simulink library "pwrsysVICtrl_202301"  (R2018a)
settings: Solver=VariableStepAuto  StartTime=0.0  StopTime=10.0  RelTol=1e-3
values from neighbouring files (symbols this model uses):
  Ts = 1e-6    (= 1e-06)    [SequenceSeparation_script.m]
undefined symbols (not defined in the file or in its folder): fn, Kp, Ti, Ts_control, Uabp, WT, X, zeta
libraries: pwrsysBasic x12, powerlib_meascontrol x8, pwrsysVICtrl x5, pwrsysTransf x1
settings Model: Creator=daniemot  LastModifiedBy=daniemot
settings OptimizationCC: LifeSpan=inf
settings DebuggingCC: SFExecutionAtInitializationDiag=none
settings CodeAppCC: StateflowObjectComments=on

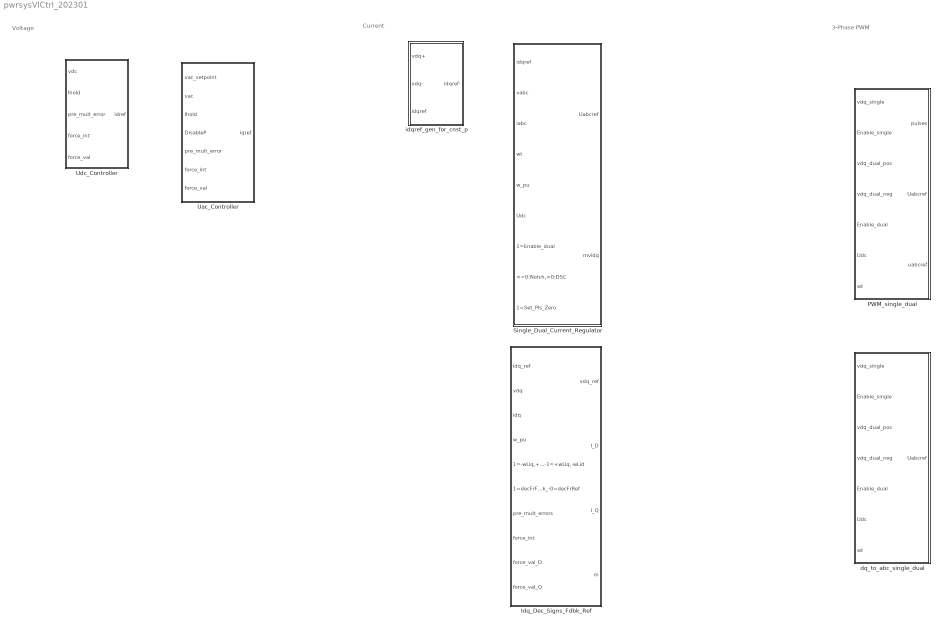
== system pwrsysVICtrl_202301 ==
  note: Voltage
  note: Current
  note: 3-Phase PWM
  Idq_Dec_Signs_Fdbk_Ref : Subsystem  mask(Idq Controller - PI regulator with anti-windup){Ts=Ts_control, fn=50, Kp=0.4, Ti=0.13, L=0.3, PI_max=1.5, PI_min=-1.5, TrafoPhaseComp=0}
      mask prompts: Ts "Sampling time [s]"; fn "Rated frequency: fn [Hz]"; Kp "Proportional gain: Kp [pu]"; Ti "Integral time: Ti [s]"; L "DQ decoupl. inductance: L [pu]"; PI_max "Maximum output [pu]"; PI_min "Minimum output [pu]"; TrafoPhaseComp "Transformer phase compensation [rad]"
      mask help:
      | Idq Controller
      | Discrete PI regulator with forward Euler approximation for the integrator.
      | Transfer function: 	Kp (1 + sTi) / (sTi)
      | The anti-windup freezes the integrator if the unlimited output of the PI goes beyond the limits.
      |
      | Phase compensation for transformer winding: PhaseTrafoComp
  PWM_single_dual : Subsystem  mask(Scaling of vdq ref and PWM gate generation){fsw=50, Ts=1/200000, Uabp=1000, PWM_Ini_Phase=90}
      mask prompts: fsw "Switching frequency [Hz]"; Ts "Sampling time [s]"; Uabp "Rated peak line voltage [V]"; PWM_Ini_Phase "PWM carrier initial phase [degrees]"
      mask help:
      | Scales vdq_ref by: U_line_peak / Udc
      |
      | Add third harmonic to uabc_ref for overmodulation
  Single_Dual_Current_Regulator : Subsystem  mask(Notch based dual dq current regulator){Ts=Ts_control, fgrid=fn, PI_X=X, PI_max=1.5, PI_min=-1.5, PWM_Uabp=Uabp, zetanotch=zeta, flpf=zeta, PI_Kp_single=Kp, PI_Ti_single=Ti, PI_Kp_dual=Kp, PI_Ti_dual=Ti}
      mask prompts: Ts "Sampling time controller [s]"; fgrid "Grid frequency [Hz]"; PI_X "Decoupling reactance X [pu]"; PI_max "PI max [pu]"; PI_min "PI min [pu]"; PWM_Uabp "Rated peak line voltage [V]"; zetanotch "Damping notch filters"; flpf "Cut-out frequelcy LPF noise [Hz]"; PI_Kp_single "Proportional gain Kp [pu/pu]"; PI_Ti_single "Integrator time Ti [s]"; PI_Kp_dual "Proportional gain Kp [pu/pu]"; PI_Ti_dual "Integrator time Ti [s]"
      mask help: To be used with "abc -> dq" and "acb -> dq" transformations. When va = V sin (wt), vb = V sin (wt-120), vc = V sin (wt+120), -> vd = V vq=0.
      mask DialogControl Container2 Prompt: Transducers
      mask DialogControl Container7 Prompt: PI regulator - Single
      mask DialogControl Container7_copy Prompt: PI regulator - Dual
  Uac_Controller : Subsystem  mask(Udc Controller - PI regulator with anti-windup){Ts=Ts_control, Kg=1, Kp=WT.LSC.Kp, Ti=WT.LSC.Ti, PI_max=1.5, PI_min=-1.5}
      mask prompts: Ts "Sampling time [s]"; Kg "Loop gain: Kg [pu]"; Kp "Proportional gain: Kp [pu]"; Ti "Integral time: Ti [s]"; PI_max "Maximum output [pu]"; PI_min "Minimum output [pu]"
      mask help:
      | Udc Controller
      | Discrete PI regulator with forward Euler approximation for the integrator.
      | Transfer function: 	Kp (1 + sTi) / (sTi)
      | The anti-windup freezes the integrator if the unlimited output of the PI goes beyond the limits.
  Udc_Controller : Subsystem  mask(Udc Controller - PI regulator with anti-windup){Ts=Ts_control, Kp=WT.LSC.Kp, Ti=WT.LSC.Ti, PI_max=1.5, PI_min=-1.5}
      mask prompts: Ts "Sampling time [s]"; Kp "Proportional gain: Kp [pu]"; Ti "Integral time: Ti [s]"; PI_max "Maximum output [pu]"; PI_min "Minimum output [pu]"
      mask help:
      | Udc Controller
      | Discrete PI regulator with forward Euler approximation for the integrator.
      | Transfer function: 	Kp (1 + sTi) / (sTi)
      | The anti-windup freezes the integrator if the unlimited output of the PI goes beyond the limits.
  dq_to_abc_single_dual : Subsystem  mask(Scaling of vdq ref and PWM gate generation){Ts=1/200000, Uabp=1000}
      mask prompts: Ts "Sampling time [s]"; Uabp "Rated peak line voltage [V]"
      mask help:
      | Scales vdq_ref by: U_line_peak / Udc
      |
      | Add third harmonic to uabc_ref for overmodulation
  idqref_gen_for_cnst_p : Subsystem  mask(Negative sequence current reference calculation){Ts_control=Ts_control}
      mask prompts: Ts_control "Sampling time [s]"
      mask help: Calculation of the negative sequence current references for removing active power second harmonic oscillations when in the presence of unbalanced voltages.
      mask Help:
      | Calculation of the negative sequence current references for removing active power second harmonic oscillations when in the presence of unbalanced voltages.
      | 
      | Second harmonic in instataneous reactive power will be increased as a result of the removal of the second harmonic in the active power.
      | 
      | To be used with "abc -> dq" and "acb -> dq" transformations. When va = V sin (wt), vb = V sin (wt-120), vc = V sin (wt+120), -> vd = V vq=0.
      | 
      | In "expanded" matrix form:
      | 	| idn | = - | -vdp  +vqp |^{-1} * | -vdn  +vqn | * | idp |
      | 	| iqn | =   | +vqp  +vdp |        | +vqn  +vdn |   | idq |
      | 
      | In matrix form
      | 	idqn  = - vdqp^{-1} * vdqn * idqp
      | 
      | Derived independently from, but later noticed that it was proposed by Chaudhary in 2012 at "Negative Sequence Current Control in Wind Power Plants With VSC-HVDC Connection", see eq. (11).
      | 
      | This block does not work for "abc (-omega) -> dq" (the formulation of Chaudhary 2012).

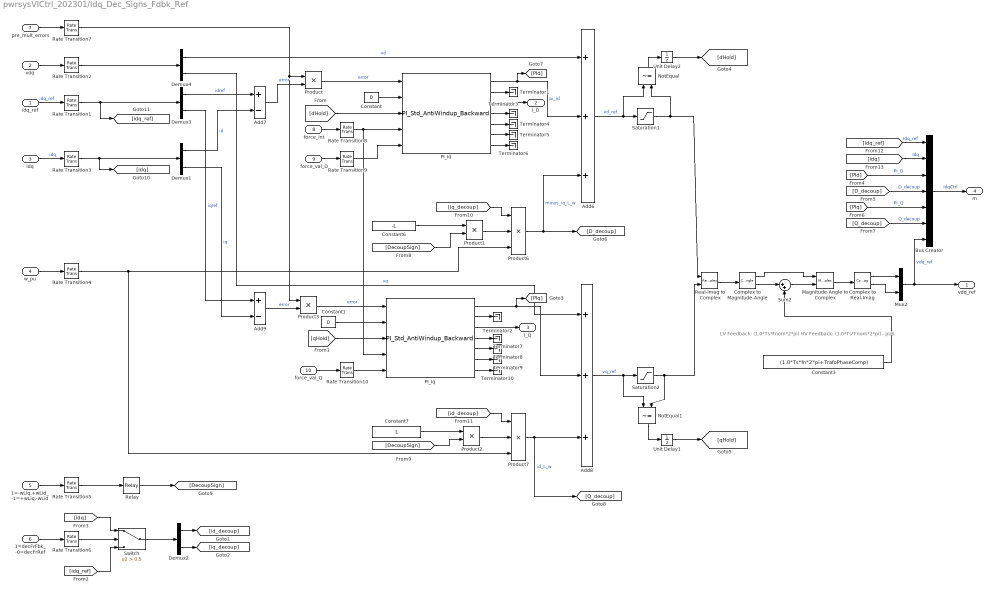
== system pwrsysVICtrl_202301/Idq_Dec_Signs_Fdbk_Ref ==
  note: LV Feedback: (1.0*Ts*Fnom*2*pi)
      | HV Feedback: (1.0*Ts*Fnom*2*pi) - pi/6
  idq_ref : Inport
  vdq : Inport  Port=2
  idq : Inport  Port=3
  w_pu : Inport  Port=4
  1=-wLiq,+wLid_-1=+wLiq,-wLid : Inport  Port=5
  1=decFrFbk_-0=decFrRef : Inport  Port=6
  pre_mult_errors : Inport  Port=7
  force_int : Inport  Port=8
  force_val_D : Inport  Port=9
  force_val_Q : Inport  Port=10
  Add6 : Sum  Inputs=+++
  Add7 : Sum  Inputs=+-
  Add8 : Sum  Inputs=+++
  Add9 : Sum  Inputs=+-
  Bus Creator : BusCreator  Inputs=7
  Complex to Magnitude-Angle : ComplexToMagnitudeAngle
  Complex to Real-Imag : ComplexToRealImag
  Constant : Constant  Value=0  SampleTime=Ts
  Constant1 : Constant  Value=0  SampleTime=Ts
  Constant3 : Constant  Value=(1.0*Ts*fn*2*pi+TrafoPhaseComp)  SampleTime=Ts
  Constant6 : Constant  Value=-L  SampleTime=Ts
  Constant7 : Constant  Value=L  SampleTime=Ts
  Demux{1..4} (4 alike) : Demux  Outputs=2
  Magnitude-Angle to Complex : MagnitudeAngleToComplex
  Mux2 : Mux  Inputs=2
  NotEqual : RelationalOperator  Operator=~=  OutDataTypeStr=boolean  RndMeth=Nearest
  NotEqual1 : RelationalOperator  Operator=~=  OutDataTypeStr=boolean  RndMeth=Nearest
  PI_Id : pwrsysBasic/PI_Std_AntiWindup_Backward  Ts=Ts  Kg=Kp  Kp=1  Ti=Ti  outMax=PI_max  outMin=PI_min
      settings: SourceProductName=NTNU Power Systems
  PI_Iq : pwrsysBasic/PI_Std_AntiWindup_Backward  Ts=Ts  Kg=Kp  Kp=1  Ti=Ti  outMax=PI_max  outMin=PI_min
      settings: SourceProductName=NTNU Power Systems
  Product : Product
  Product1 : Product  RndMeth=Zero
  Product2 : Product  RndMeth=Zero
  Product3 : Product
  Product6 : Product  Inputs=3  RndMeth=Zero
  Product7 : Product  Inputs=3  RndMeth=Zero
  Rate Transition1 : RateTransition  InitialCondition=[0 0]  OutPortSampleTime=Ts
  Rate Transition{6..10} (5 alike) : RateTransition  OutPortSampleTime=Ts
  Rate Transition2 : RateTransition  InitialCondition=[0 0]  OutPortSampleTime=Ts
  Rate Transition3 : RateTransition  InitialCondition=[0 0]  OutPortSampleTime=Ts
  Rate Transition4 : RateTransition  InitialCondition=1  OutPortSampleTime=Ts
  Rate Transition5 : RateTransition  InitialCondition=1  OutPortSampleTime=Ts
  Real-Imag to Complex : RealImagToComplex
  Relay : Relay  OnSwitchValue=0  OffSwitchValue=-0.1  OffOutputValue=-1
  Saturation1 : Saturate  UpperLimit=PI_max  LowerLimit=PI_min
  Saturation2 : Saturate  UpperLimit=PI_max  LowerLimit=PI_min
  Sum2 : Sum  Inputs=|++
  Switch : Switch  Criteria=u2 > Threshold  Threshold=0.5
  Terminator{1..10} (10 alike) : Terminator
  Unit Delay1 : UnitDelay  SampleTime=Ts
  Unit Delay2 : UnitDelay  SampleTime=Ts
  vdq_ref : Outport
  I_D : Outport  Port=2
  I_Q : Outport  Port=3
  m : Outport  Port=4
  wires:
  w_pu/1 -> Rate Transition4/1
  Product3/1 -> PI_Iq/1  "error"
  PI_Id/1 -> Add6/2, [PId]  "pi_id"
  Constant6/1 -> Product1/1
  Constant7/1 -> Product2/1
  Demux1/1 -> Add7/2  "id"
  Product7/1 -> [Q_decoup], Add8/3  "id_L_w"
  Demux4/1 -> Add6/1  "vd"
  Product/1 -> PI_Id/1  "error"
  Demux1/2 -> Add9/2  "iq"
  Product6/1 -> Add6/3, [D_decoup]  "minus_iq_L_w"
  Demux4/2 -> Add8/1  "vq"
  Mux2/1 -> Bus Creator/7, vdq_ref/1  "vdq_ref"
  idq/1 -> Rate Transition3/1  "idq"
  vdq/1 -> Rate Transition2/1
  Add8/1 -> NotEqual1/1, Saturation2/1  "vq_ref"
  Add6/1 -> NotEqual/1, Saturation1/1  "vd_ref"
  idq_ref/1 -> Rate Transition1/1  "idq_ref"
  Demux3/1 -> Add7/1  "idref"
  Demux3/2 -> Add9/1  "iqref"
  Magnitude-Angle to Complex/1 -> Complex to Real-Imag/1
  Real-Imag to Complex/1 -> Complex to Magnitude-Angle/1
  Complex to Magnitude-Angle/1 -> Magnitude-Angle to Complex/1
  Complex to Magnitude-Angle/2 -> Sum2/1
  Sum2/1 -> Magnitude-Angle to Complex/2
  Constant3/1 -> Sum2/2
  Complex to Real-Imag/1 -> Mux2/1
  Complex to Real-Imag/2 -> Mux2/2
  [PId] -> Bus Creator/3  "PI_D"
  [D_decoup] -> Bus Creator/4  "D_decoup"
  [PIq] -> Bus Creator/5  "PI_Q"
  Bus Creator/1 -> m/1  "IdqCtrl"
  [Q_decoup] -> Bus Creator/6  "Q_decoup"
  Saturation1/1 -> NotEqual/2, Real-Imag to Complex/1
  NotEqual/1 -> Unit Delay2/1
  Saturation2/1 -> NotEqual1/2, Real-Imag to Complex/2
  NotEqual1/1 -> Unit Delay1/1
  Unit Delay2/1 -> [dHold]
  Unit Delay1/1 -> [qHold]
  [dHold] -> PI_Id/3
  [qHold] -> PI_Iq/3
  Relay/1 -> [DecoupSign]
  1=-wLiq,+wLid_-1=+wLiq,-wLid/1 -> Rate Transition5/1
  [DecoupSign] -> Product1/2
  Product1/1 -> Product6/2
  Product2/1 -> Product7/2
  [DecoupSign] -> Product2/2
  [idq_ref] -> Switch/3
  Demux2/2 -> [iq_decoup]
  1=decFrFbk_-0=decFrRef/1 -> Rate Transition6/1
  Demux2/1 -> [id_decoup]
  Switch/1 -> Demux2/1
  [idq] -> Switch/1
  [iq_decoup] -> Product6/1
  [id_decoup] -> Product7/1
  [idq_ref] -> Bus Creator/1  "Idq_ref"
  [idq] -> Bus Creator/2  "Idq"
  force_int/1 -> Rate Transition8/1
  force_val_D/1 -> Rate Transition9/1
  force_val_Q/1 -> Rate Transition10/1
  Add9/1 -> Product3/2  "error"
  Add7/1 -> Product/2  "error"
  pre_mult_errors/1 -> Rate Transition7/1
  PI_Id/3 -> I_D/1
  Constant/1 -> PI_Id/2
  PI_Id/2 -> Terminator1/1
  PI_Id/4 -> Terminator3/1
  PI_Id/5 -> Terminator4/1
  PI_Id/6 -> Terminator5/1
  PI_Id/7 -> Terminator6/1
  PI_Iq/2 -> Terminator2/1
  PI_Iq/4 -> Terminator7/1
  PI_Iq/5 -> Terminator8/1
  PI_Iq/6 -> Terminator9/1
  PI_Iq/7 -> Terminator10/1
  PI_Iq/3 -> I_Q/1
  PI_Iq/1 -> Add8/2, [PIq]
  Constant1/1 -> PI_Iq/2
  Rate Transition2/1 -> Demux4/1
  Rate Transition1/1 -> [idq_ref], Demux3/1
  Rate Transition3/1 -> Demux1/1, [idq]
  Rate Transition4/1 -> Product7/3, Product6/3
  Rate Transition5/1 -> Relay/1
  Rate Transition6/1 -> Switch/2
  Rate Transition7/1 -> Product3/1, Product/1
  Rate Transition8/1 -> PI_Iq/4, PI_Id/4
  Rate Transition9/1 -> PI_Id/5
  Rate Transition10/1 -> PI_Iq/5

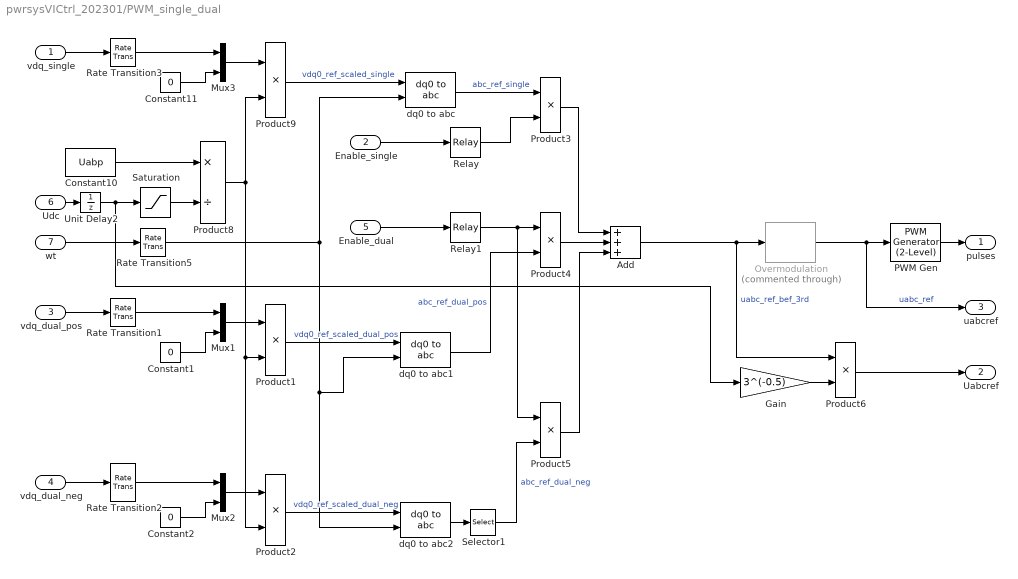
== system pwrsysVICtrl_202301/PWM_single_dual ==
  vdq_single : Inport
  Enable_single : Inport  Port=2
  vdq_dual_pos : Inport  Port=3
  vdq_dual_neg : Inport  Port=4
  Enable_dual : Inport  Port=5
  Udc : Inport  Port=6
  wt : Inport  Port=7
  Add : Sum  Inputs=+++
  Constant1 : Constant  Value=0
  Constant10 : Constant  Value=Uabp
  Constant11 : Constant  Value=0
  Constant2 : Constant  Value=0
  Gain : Gain  Gain=3^(-0.5)
  Mux1 : Mux  Inputs=[2 1]
  Mux2 : Mux  Inputs=[2 1]
  Mux3 : Mux  Inputs=[2 1]
  Overmodulation : powerlib_meascontrol/Pulse & Signal Generators/Overmodulation  Commented=through  OverModType=Third harmonic
      settings: SourceProductName=Simscape Power Systems  SourceProductBaseCode=PS
  PWM Gen : powerlib_meascontrol/Pulse & Signal Generators/PWM Generator (2-Level)  ModulatorType=Three-phase bridge (6 pulses)  ModulatorMode=Unsynchronized  Fc=fsw  Pc=PWM_Ini_Phase  nF=27  MinMax="[ -1  1 ]"  SamplingTechnique=Asymmetrical regular (double edge)  ModulatingSignals=off  m=0.8  Freq=60  Phase=0  Ts=Ts  ShowCarrierOutport=off
      settings: SourceProductName=Simscape Power Systems
  Product{1..6,9} (7 alike) : Product  Inputs=**
  Product8 : Product  Inputs=*/
  Rate Transition{1..3,5} (4 alike) : RateTransition  OutPortSampleTime=Ts
  Relay : Relay  OnSwitchValue=0.6  OffSwitchValue=0.4
  Relay1 : Relay  OnSwitchValue=0.6  OffSwitchValue=0.4
  Saturation : Saturate  UpperLimit=10*Uabp  LowerLimit=0.001*Uabp
  Selector1 : Selector  InputPortWidth=3  IndexOptions=Index vector (dialog)  Indices=[1 3 2]  OutputSizes=1
  Unit Delay2 : UnitDelay  InitialCondition=Uabp  SampleTime=Ts
  dq0 to abc : powerlib_meascontrol/Transformations/dq0 to abc  Alignment=90 degrees behind phase A axis
  dq0 to abc1 : powerlib_meascontrol/Transformations/dq0 to abc  Alignment=90 degrees behind phase A axis
  dq0 to abc2 : powerlib_meascontrol/Transformations/dq0 to abc  Alignment=90 degrees behind phase A axis
  pulses : Outport
  Uabcref : Outport  Port=2
  uabcref : Outport  Port=3
  wires:
  dq0 to abc1/1 -> Product4/2  "abc_ref_dual_pos"
  Rate Transition5/1 -> dq0 to abc/2, dq0 to abc1/2, dq0 to abc2/2
  Product1/1 -> dq0 to abc1/1  "vdq0_ref_scaled_dual_pos"
  vdq_dual_pos/1 -> Rate Transition1/1
  Constant1/1 -> Mux1/2
  Mux1/1 -> Product1/1
  Rate Transition1/1 -> Mux1/1
  Product6/1 -> Uabcref/1
  vdq_single/1 -> Rate Transition3/1
  PWM Gen/1 -> pulses/1
  Udc/1 -> Unit Delay2/1
  Overmodulation/1 -> uabcref/1, PWM Gen/1  "uabc_ref"
  Constant10/1 -> Product8/1
  wt/1 -> Rate Transition5/1
  Rate Transition3/1 -> Mux3/1
  Mux3/1 -> Product9/1
  Unit Delay2/1 -> Gain/1, Saturation/1
  Product9/1 -> dq0 to abc/1  "vdq0_ref_scaled_single"
  Constant11/1 -> Mux3/2
  dq0 to abc/1 -> Product3/1  "abc_ref_single"
  Enable_single/1 -> Relay/1
  Enable_dual/1 -> Relay1/1
  Add/1 -> Product6/1, Overmodulation/1  "uabc_ref_bef_3rd"
  Saturation/1 -> Product8/2
  Product8/1 -> Product2/2, Product1/2, Product9/2
  Rate Transition2/1 -> Mux2/1
  vdq_dual_neg/1 -> Rate Transition2/1
  Mux2/1 -> Product2/1
  Constant2/1 -> Mux2/2
  Product2/1 -> dq0 to abc2/1  "vdq0_ref_scaled_dual_neg"
  dq0 to abc2/1 -> Selector1/1
  Selector1/1 -> Product5/2  "abc_ref_dual_neg"
  Relay/1 -> Product3/2
  Product3/1 -> Add/1
  Product4/1 -> Add/2
  Relay1/1 -> Product5/1, Product4/1
  Product5/1 -> Add/3
  Gain/1 -> Product6/2

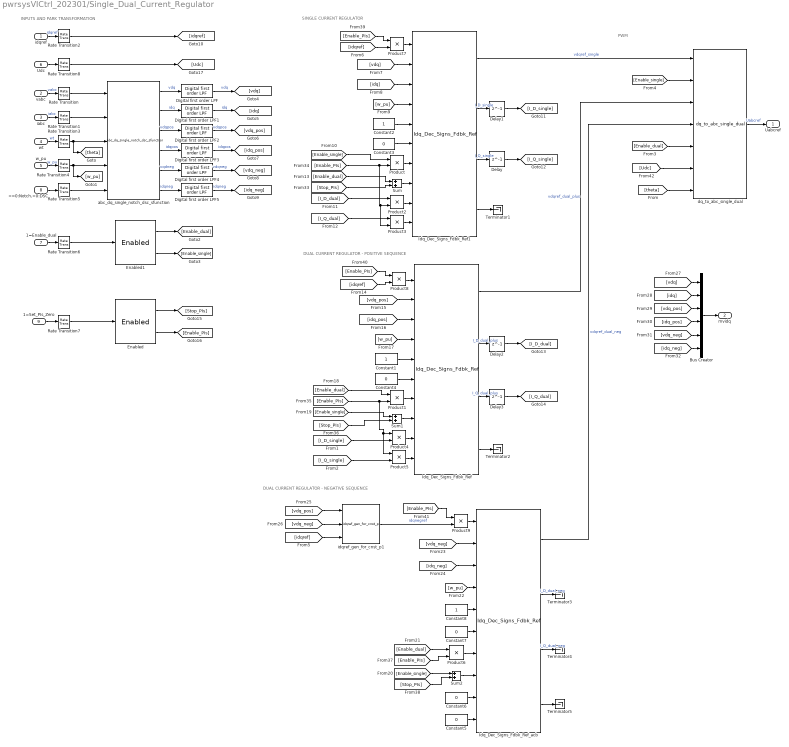
== system pwrsysVICtrl_202301/Single_Dual_Current_Regulator ==
  note: INPUTS AND PARK TRANSFORMATION
  note: SINGLE CURRENT REGULATOR
  note: DUAL CURRENT REGULATOR - POSITIVE SEQUENCE
  note: DUAL CURRENT REGULATOR - NEGATIVE SEQUENCE
  note: PWM
  idqref : Inport
  vabc : Inport  Port=2
  iabc : Inport  Port=3
  wt : Inport  Port=4
  w_pu : Inport  Port=5
  Udc : Inport  Port=6
  1=Enable_dual : Inport  Port=7
  <=0:Notch,>0:DSC : Inport  Port=8
  1=Set_PIs_Zero : Inport  Port=9
  Bus Creator : BusCreator  Inputs=6
  Constant1 : Constant  SampleTime=Ts
  Constant2 : Constant  SampleTime=Ts
  Constant{3..7} (5 alike) : Constant  Value=0  SampleTime=Ts
  Constant8 : Constant  SampleTime=Ts
  Delay{,1..3} (4 alike) : Delay  DelayLength=1  InitialCondition=0  SampleTime=Ts
  Digital first order LPF{,1..5} (6 alike) : pwrsysBasic/Digital first order LPF  Ts=Ts  fcutout=flpf
      settings: SourceProductName=NTNU Power Systems
  Enabled : pwrsysBasic/Enabled
      settings: SourceProductName=NTNU Power Systems
  Enabled1 : pwrsysBasic/Enabled
      settings: SourceProductName=NTNU Power Systems
  Idq_Dec_Signs_Fdbk_Ref : pwrsysVICtrl/Idq_Dec_Signs_Fdbk_Ref  Ts=Ts  fn=fgrid  Kp=PI_Kp_dual  Ti=PI_Ti_dual  L=PI_X  PI_max=PI_max  PI_min=PI_min  TrafoPhaseComp=0
      settings: SourceProductName=NTNU Power Systems
  Idq_Dec_Signs_Fdbk_Ref1 : pwrsysVICtrl/Idq_Dec_Signs_Fdbk_Ref  Ts=Ts  fn=fgrid  Kp=PI_Kp_single  Ti=PI_Ti_single  L=PI_X  PI_max=PI_max  PI_min=PI_min  TrafoPhaseComp=0
      settings: SourceProductName=NTNU Power Systems
  Idq_Dec_Signs_Fdbk_Ref_acb : pwrsysVICtrl/Idq_Dec_Signs_Fdbk_Ref  Ts=Ts  fn=fgrid  Kp=PI_Kp_dual  Ti=PI_Ti_dual  L=PI_X  PI_max=PI_max  PI_min=PI_min  TrafoPhaseComp=0
      settings: SourceProductName=NTNU Power Systems
  Product{,1..9} (10 alike) : Product
  Rate Transition : RateTransition  InitialCondition=[0 0 0]  OutPortSampleTime=Ts
  Rate Transition1 : RateTransition  InitialCondition=[0 0 0]  OutPortSampleTime=Ts
  Rate Transition2 : RateTransition  InitialCondition=[0 0]  OutPortSampleTime=Ts
  Rate Transition{3,5..7} (4 alike) : RateTransition  OutPortSampleTime=Ts
  Rate Transition4 : RateTransition  InitialCondition=1  OutPortSampleTime=Ts
  Rate Transition8 : RateTransition  InitialCondition=1  OutPortSampleTime=Ts
  Sum : Sum
  Sum1 : Sum
  Sum2 : Sum
  Terminator{1..5} (5 alike) : Terminator
  abc_dq_single_notch_dsc_sfunction : pwrsysTransf/abc_dq_single_notch_dsc_sfunction  Ts=Ts  fn=2*fgrid  zeta=zetanotch
      settings: SourceProductName=NTNU Power Systems
  dq_to_abc_single_dual : pwrsysVICtrl/dq_to_abc_single_dual  Ts=Ts  Uabp=PWM_Uabp
      settings: SourceProductName=NTNU Power Systems
  idqref_gen_for_cnst_p1 : pwrsysVICtrl/idqref_gen_for_cnst_p  Ts_control=Ts
      settings: SourceProductName=NTNU Power Systems
  Uabcref : Outport
  mvidq : Outport  Port=2
  wires:
  1=Enable_dual/1 -> Rate Transition6/1
  Enabled1/2 -> [Enable_single]
  Enabled1/1 -> [Enable_dual]
  1=Set_PIs_Zero/1 -> Rate Transition7/1
  Product9/1 -> Idq_Dec_Signs_Fdbk_Ref_acb/1
  [Enable_PIs] -> Product9/1
  Product8/1 -> Idq_Dec_Signs_Fdbk_Ref/1
  [Enable_PIs] -> Product8/1
  Product7/1 -> Idq_Dec_Signs_Fdbk_Ref1/1
  [Enable_PIs] -> Product7/1
  Sum2/1 -> Idq_Dec_Signs_Fdbk_Ref_acb/8
  [Stop_PIs] -> Sum2/2
  Product6/1 -> Idq_Dec_Signs_Fdbk_Ref_acb/7
  [Enable_PIs] -> Product6/2
  Product4/1 -> Idq_Dec_Signs_Fdbk_Ref/9
  Product5/1 -> Idq_Dec_Signs_Fdbk_Ref/10
  [Stop_PIs] -> Sum1/2
  Sum1/1 -> Idq_Dec_Signs_Fdbk_Ref/8
  [Enable_PIs] -> Product1/2, Product4/1, Product5/1
  Product1/1 -> Idq_Dec_Signs_Fdbk_Ref/7
  Product2/1 -> Idq_Dec_Signs_Fdbk_Ref1/9
  [Stop_PIs] -> Sum/2
  Product3/1 -> Idq_Dec_Signs_Fdbk_Ref1/10
  Sum/1 -> Idq_Dec_Signs_Fdbk_Ref1/8
  Product/1 -> Idq_Dec_Signs_Fdbk_Ref1/7
  [Enable_PIs] -> Product/2, Product2/2, Product3/2
  Enabled/2 -> [Enable_PIs]
  Enabled/1 -> [Stop_PIs]
  [idq_neg] -> Bus Creator/6
  [vdq_neg] -> Bus Creator/5
  [idq_pos] -> Bus Creator/4
  [vdq_pos] -> Bus Creator/3
  [idq] -> Bus Creator/2
  [vdq] -> Bus Creator/1
  Bus Creator/1 -> mvidq/1
  Idq_Dec_Signs_Fdbk_Ref_acb/1 -> dq_to_abc_single_dual/4  "vdqref_dual_neg"
  Idq_Dec_Signs_Fdbk_Ref/1 -> dq_to_abc_single_dual/3  "vdqref_dual_plus"
  Idq_Dec_Signs_Fdbk_Ref1/1 -> dq_to_abc_single_dual/1  "vdqref_single"
  idqref_gen_for_cnst_p1/1 -> Product9/2  "idqnegref"
  [vdq_neg] -> idqref_gen_for_cnst_p1/2
  [vdq_pos] -> idqref_gen_for_cnst_p1/1
  [idq_neg] -> Idq_Dec_Signs_Fdbk_Ref_acb/3
  [vdq_neg] -> Idq_Dec_Signs_Fdbk_Ref_acb/2
  [w_pu] -> Idq_Dec_Signs_Fdbk_Ref_acb/4
  Constant8/1 -> Idq_Dec_Signs_Fdbk_Ref_acb/5
  Constant7/1 -> Idq_Dec_Signs_Fdbk_Ref_acb/6
  [Enable_dual] -> Product6/1
  [Enable_single] -> Sum2/1
  Constant6/1 -> Idq_Dec_Signs_Fdbk_Ref_acb/9
  Constant5/1 -> Idq_Dec_Signs_Fdbk_Ref_acb/10
  Idq_Dec_Signs_Fdbk_Ref_acb/4 -> Terminator5/1
  Idq_Dec_Signs_Fdbk_Ref_acb/3 -> Terminator4/1  "I_Q_dual_neg"
  Idq_Dec_Signs_Fdbk_Ref_acb/2 -> Terminator3/1  "I_D_dual_neg"
  Idq_Dec_Signs_Fdbk_Ref/4 -> Terminator2/1
  Idq_Dec_Signs_Fdbk_Ref1/4 -> Terminator1/1
  [Enable_single] -> Sum1/1
  [Enable_dual] -> Product1/1
  Constant4/1 -> Idq_Dec_Signs_Fdbk_Ref/6
  Constant1/1 -> Idq_Dec_Signs_Fdbk_Ref/5
  [w_pu] -> Idq_Dec_Signs_Fdbk_Ref/4
  [idq_pos] -> Idq_Dec_Signs_Fdbk_Ref/3
  [vdq_pos] -> Idq_Dec_Signs_Fdbk_Ref/2
  [idqref] -> Product8/2
  [Enable_dual] -> Sum/1
  [I_Q_dual] -> Product3/1
  [I_D_dual] -> Product2/1
  [I_Q_single] -> Product5/2
  [I_D_single] -> Product4/2
  Delay3/1 -> [I_Q_dual]
  Delay2/1 -> [I_D_dual]
  Delay/1 -> [I_Q_single]
  Delay1/1 -> [I_D_single]
  Idq_Dec_Signs_Fdbk_Ref/3 -> Delay3/1  "I_Q_dual_plus"
  Idq_Dec_Signs_Fdbk_Ref/2 -> Delay2/1  "I_D_dual_plus"
  Idq_Dec_Signs_Fdbk_Ref1/2 -> Delay1/1  "I_D_single"
  Idq_Dec_Signs_Fdbk_Ref1/3 -> Delay/1  "I_Q_single"
  [Enable_single] -> Product/1
  <=0:Notch,>0:DSC/1 -> Rate Transition5/1
  Constant3/1 -> Idq_Dec_Signs_Fdbk_Ref1/6
  Constant2/1 -> Idq_Dec_Signs_Fdbk_Ref1/5
  [w_pu] -> Idq_Dec_Signs_Fdbk_Ref1/4
  [idq] -> Idq_Dec_Signs_Fdbk_Ref1/3
  [vdq] -> Idq_Dec_Signs_Fdbk_Ref1/2
  [idqref] -> Product7/2
  idqref/1 -> Rate Transition2/1  "idqref"
  w_pu/1 -> Rate Transition4/1  "w_pu"
  wt/1 -> Rate Transition3/1  "wt"
  iabc/1 -> Rate Transition1/1  "iabc"
  vabc/1 -> Rate Transition/1  "vabc"
  [Enable_single] -> dq_to_abc_single_dual/2
  [Enable_dual] -> dq_to_abc_single_dual/5
  [theta] -> dq_to_abc_single_dual/7
  [idqref] -> idqref_gen_for_cnst_p1/3
  dq_to_abc_single_dual/1 -> Uabcref/1  "Uabcref"
  abc_dq_single_notch_dsc_sfunction/1 -> Digital first order LPF/1  "vdq"
  abc_dq_single_notch_dsc_sfunction/2 -> Digital first order LPF1/1  "idq"
  abc_dq_single_notch_dsc_sfunction/3 -> Digital first order LPF2/1  "vdqpos"
  abc_dq_single_notch_dsc_sfunction/4 -> Digital first order LPF3/1  "idqpos"
  abc_dq_single_notch_dsc_sfunction/5 -> Digital first order LPF4/1  "vqdneg"
  abc_dq_single_notch_dsc_sfunction/6 -> Digital first order LPF5/1  "idqneg"
  Rate Transition/1 -> abc_dq_single_notch_dsc_sfunction/1
  Rate Transition1/1 -> abc_dq_single_notch_dsc_sfunction/2
  Rate Transition2/1 -> [idqref]
  Rate Transition3/1 -> abc_dq_single_notch_dsc_sfunction/3, [theta]
  Rate Transition4/1 -> abc_dq_single_notch_dsc_sfunction/4, [w_pu]
  Rate Transition5/1 -> abc_dq_single_notch_dsc_sfunction/5
  Rate Transition6/1 -> Enabled1/1
  Rate Transition7/1 -> Enabled/1
  [Udc] -> dq_to_abc_single_dual/6
  Udc/1 -> Rate Transition8/1
  Rate Transition8/1 -> [Udc]
  Digital first order LPF/1 -> [vdq]  "vdq"
  Digital first order LPF1/1 -> [idq]  "idq"
  Digital first order LPF2/1 -> [vdq_pos]  "vdqpos"
  Digital first order LPF3/1 -> [idq_pos]  "idqpos"
  Digital first order LPF4/1 -> [vdq_neg]  "vdqneg"
  Digital first order LPF5/1 -> [idq_neg]  "idqneg"

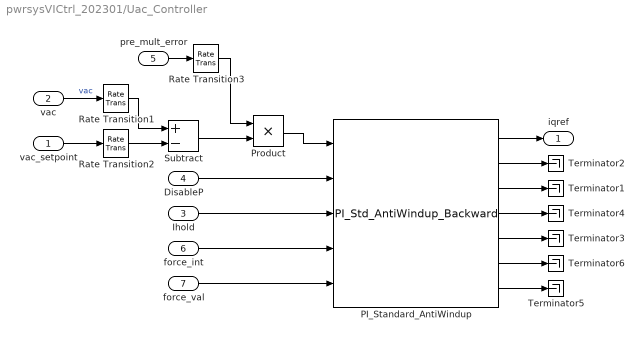
== system pwrsysVICtrl_202301/Uac_Controller ==
  vac_setpoint : Inport
  vac : Inport  Port=2
  Ihold : Inport  Port=3
  DisableP : Inport  Port=4
  pre_mult_error : Inport  Port=5
  force_int : Inport  Port=6
  force_val : Inport  Port=7
  PI_Standard_AntiWindup : pwrsysBasic/PI_Std_AntiWindup_Backward  Ts=Ts  Kg=Kg  Kp=Kp  Ti=Ti  outMax=PI_max  outMin=PI_min
      settings: SourceProductName=NTNU Power Systems
  Product : Product
  Rate Transition1 : RateTransition  InitialCondition=1  OutPortSampleTime=Ts
  Rate Transition2 : RateTransition  InitialCondition=1  OutPortSampleTime=Ts
  Rate Transition3 : RateTransition  OutPortSampleTime=Ts
  Subtract : Sum  Inputs=+-
  Terminator{1..6} (6 alike) : Terminator
  iqref : Outport
  wires:
  vac/1 -> Rate Transition1/1  "vac"
  Subtract/1 -> Product/2
  Rate Transition1/1 -> Subtract/1
  Rate Transition2/1 -> Subtract/2
  vac_setpoint/1 -> Rate Transition2/1
  pre_mult_error/1 -> Rate Transition3/1
  Rate Transition3/1 -> Product/1
  Product/1 -> PI_Standard_AntiWindup/1
  force_val/1 -> PI_Standard_AntiWindup/5
  PI_Standard_AntiWindup/1 -> iqref/1
  PI_Standard_AntiWindup/2 -> Terminator2/1
  PI_Standard_AntiWindup/3 -> Terminator1/1
  PI_Standard_AntiWindup/5 -> Terminator3/1
  PI_Standard_AntiWindup/4 -> Terminator4/1
  PI_Standard_AntiWindup/6 -> Terminator6/1
  PI_Standard_AntiWindup/7 -> Terminator5/1
  DisableP/1 -> PI_Standard_AntiWindup/2
  Ihold/1 -> PI_Standard_AntiWindup/3
  force_int/1 -> PI_Standard_AntiWindup/4

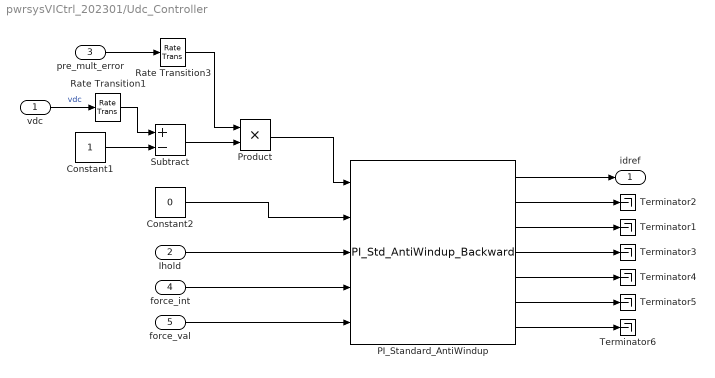
== system pwrsysVICtrl_202301/Udc_Controller ==
  vdc : Inport
  Ihold : Inport  Port=2
  pre_mult_error : Inport  Port=3
  force_int : Inport  Port=4
  force_val : Inport  Port=5
  Constant1 : Constant
  Constant2 : Constant  Value=0
  PI_Standard_AntiWindup : pwrsysBasic/PI_Std_AntiWindup_Backward  Ts=Ts  Kg=Kp  Kp=1  Ti=Ti  outMax=PI_max  outMin=PI_min
      settings: SourceProductName=NTNU Power Systems
  Product : Product
  Rate Transition1 : RateTransition  InitialCondition=1  OutPortSampleTime=Ts
  Rate Transition3 : RateTransition  OutPortSampleTime=Ts
  Subtract : Sum  Inputs=+-
  Terminator{1..6} (6 alike) : Terminator
  idref : Outport
  wires:
  vdc/1 -> Rate Transition1/1  "vdc"
  Subtract/1 -> Product/2
  Rate Transition1/1 -> Subtract/1
  Constant1/1 -> Subtract/2
  Rate Transition3/1 -> Product/1
  pre_mult_error/1 -> Rate Transition3/1
  Product/1 -> PI_Standard_AntiWindup/1
  Constant2/1 -> PI_Standard_AntiWindup/2
  PI_Standard_AntiWindup/1 -> idref/1
  PI_Standard_AntiWindup/2 -> Terminator2/1
  PI_Standard_AntiWindup/3 -> Terminator1/1
  PI_Standard_AntiWindup/4 -> Terminator3/1
  PI_Standard_AntiWindup/5 -> Terminator4/1
  PI_Standard_AntiWindup/6 -> Terminator5/1
  PI_Standard_AntiWindup/7 -> Terminator6/1
  force_val/1 -> PI_Standard_AntiWindup/5
  Ihold/1 -> PI_Standard_AntiWindup/3
  force_int/1 -> PI_Standard_AntiWindup/4

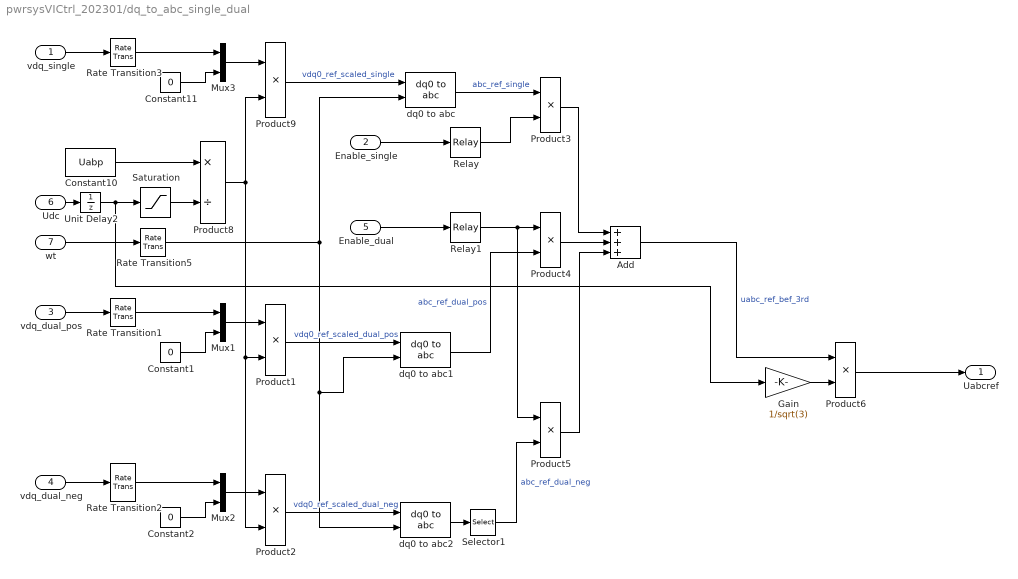
== system pwrsysVICtrl_202301/dq_to_abc_single_dual ==
  vdq_single : Inport
  Enable_single : Inport  Port=2
  vdq_dual_pos : Inport  Port=3
  vdq_dual_neg : Inport  Port=4
  Enable_dual : Inport  Port=5
  Udc : Inport  Port=6
  wt : Inport  Port=7
  Add : Sum  Inputs=+++
  Constant1 : Constant  Value=0  SampleTime=Ts
  Constant10 : Constant  Value=Uabp  SampleTime=Ts
  Constant11 : Constant  Value=0  SampleTime=Ts
  Constant2 : Constant  Value=0  SampleTime=Ts
  Gain : Gain  Gain=1/sqrt(3)
  Mux1 : Mux  Inputs=[2 1]
  Mux2 : Mux  Inputs=[2 1]
  Mux3 : Mux  Inputs=[2 1]
  Product{1..6,9} (7 alike) : Product  Inputs=**
  Product8 : Product  Inputs=*/
  Rate Transition{1..3,5} (4 alike) : RateTransition  OutPortSampleTime=Ts
  Relay : Relay  OnSwitchValue=0.6  OffSwitchValue=0.4
  Relay1 : Relay  OnSwitchValue=0.6  OffSwitchValue=0.4
  Saturation : Saturate  UpperLimit=10*Uabp  LowerLimit=0.001*Uabp
  Selector1 : Selector  InputPortWidth=3  IndexOptions=Index vector (dialog)  Indices=[1 3 2]  OutputSizes=1
  Unit Delay2 : UnitDelay  InitialCondition=Uabp  SampleTime=Ts
  dq0 to abc : powerlib_meascontrol/Transformations/dq0 to abc  Alignment=90 degrees behind phase A axis
  dq0 to abc1 : powerlib_meascontrol/Transformations/dq0 to abc  Alignment=90 degrees behind phase A axis
  dq0 to abc2 : powerlib_meascontrol/Transformations/dq0 to abc  Alignment=90 degrees behind phase A axis
  Uabcref : Outport
  wires:
  dq0 to abc1/1 -> Product4/2  "abc_ref_dual_pos"
  Rate Transition5/1 -> dq0 to abc/2, dq0 to abc1/2, dq0 to abc2/2
  Product1/1 -> dq0 to abc1/1  "vdq0_ref_scaled_dual_pos"
  vdq_dual_pos/1 -> Rate Transition1/1
  Constant1/1 -> Mux1/2
  Mux1/1 -> Product1/1
  Rate Transition1/1 -> Mux1/1
  Product6/1 -> Uabcref/1
  vdq_single/1 -> Rate Transition3/1
  Udc/1 -> Unit Delay2/1
  Constant10/1 -> Product8/1
  wt/1 -> Rate Transition5/1
  Rate Transition3/1 -> Mux3/1
  Mux3/1 -> Product9/1
  Unit Delay2/1 -> Gain/1, Saturation/1
  Product9/1 -> dq0 to abc/1  "vdq0_ref_scaled_single"
  Constant11/1 -> Mux3/2
  dq0 to abc/1 -> Product3/1  "abc_ref_single"
  Enable_single/1 -> Relay/1
  Enable_dual/1 -> Relay1/1
  Add/1 -> Product6/1  "uabc_ref_bef_3rd"
  Saturation/1 -> Product8/2
  Product8/1 -> Product2/2, Product1/2, Product9/2
  Rate Transition2/1 -> Mux2/1
  vdq_dual_neg/1 -> Rate Transition2/1
  Mux2/1 -> Product2/1
  Constant2/1 -> Mux2/2
  Product2/1 -> dq0 to abc2/1  "vdq0_ref_scaled_dual_neg"
  dq0 to abc2/1 -> Selector1/1
  Selector1/1 -> Product5/2  "abc_ref_dual_neg"
  Relay/1 -> Product3/2
  Product3/1 -> Add/1
  Product4/1 -> Add/2
  Relay1/1 -> Product5/1, Product4/1
  Product5/1 -> Add/3
  Gain/1 -> Product6/2

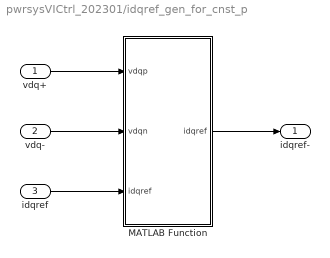
== system pwrsysVICtrl_202301/idqref_gen_for_cnst_p ==
  vdq+ : Inport
  vdq- : Inport  Port=2
  idqref : Inport  Port=3
  MATLAB Function : MATLAB Function  TreatAsAtomicUnit=on  SystemSampleTime=Ts
  idqref- : Outport
  wires:
  MATLAB Function/1(idqref) -> idqref-/1
  vdq+/1 -> MATLAB Function/1(vdqp)
  vdq-/1 -> MATLAB Function/2(vdqn)
  idqref/1 -> MATLAB Function/3("idqref ")

== matlab function pwrsysVICtrl_202301/idqref_gen_for_cnst_p/MATLAB Function ==
  data: vdqp input; idqref output; vdqn input; idqref input
function idqref = fcn(vdqp,vdqn,idqref)

% Calculation of the negative sequence references for zeroing the active 
% power second harmonic oscillations
% 
% Derived independently from, but later noticed that the same line of
% reasoning was adopted by Chaudhary 2012 "Negative Sequence Current
% Control in Wind Power Plants With VSC-HVDC Connection"

% In "expanded" matrix form
% | idn | = - | -vdp  +vqp |^{-1} * | -vdn  +vqn | * | idp | 
% | iqn | =   | +vqp  +vdp |        | +vqn  +vdn |   | idq |
% In matrix form
%  idqn   = -   vdqp^{-1}         *      vdqn      *   idqp

%The matrix that will be inverted
vp = zeros(2);
vp(1,1) = -vdqp(1);
vp(1,2) = vdqp(2);
vp(2,1) = vdqp(2);
vp(2,2) = vdqp(1);

%check is vp is invertible
if det(vp) == 0
    idqref(1,1) = 0;
    idqref(2,1) = 0;
else
    %The matrix that is not inverted
    vn = zeros(2);
    vn(1,1) = -vdqn(1);
    vn(1,2) = vdqn(2);
    vn(2,1) = vdqn(2);
    vn(2,2) = vdqn(1);

    % idqn = - vdqp^{-1} * vdqn * idqp
    idqref = -vp\vn*idqref;
end
